simulink model "SMRsimplifiedmdl"  (R2020a)
settings: Solver=VariableStepAuto  StartTime=0.0  StopTime=10.0  RelTol=1e-3
settings Model: Creator=marce  LastModifiedBy=marce

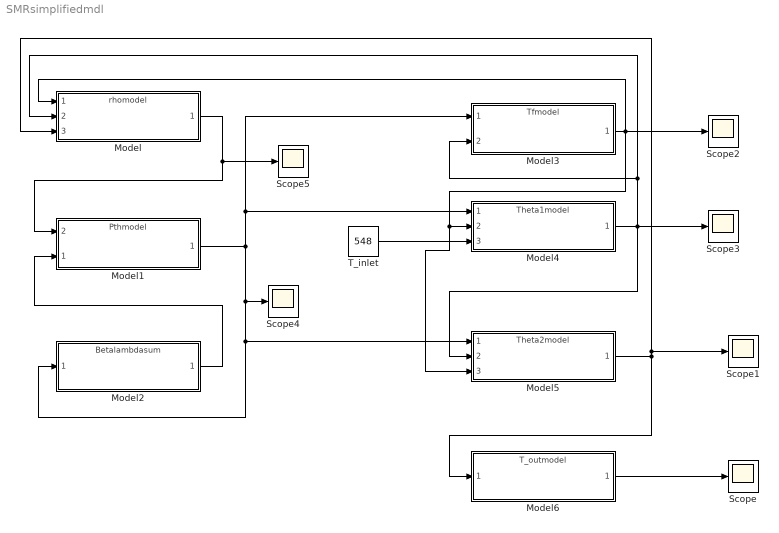
== system SMRsimplifiedmdl ==
  Model : ModelReference  ModelNameDialog=rhomodel.slx  SimulationMode=Normal  ModelReferenceVersion=1.1
  Model1 : ModelReference  ModelNameDialog=Pthmodel.slx  SimulationMode=Normal  ModelReferenceVersion=1.1
      settings: PortSchema="{\"entries\":[{\"content\":{\"sides\":[{\"content\":{\"connectorIds\":[\"In2\",\"In1\"]},\"type\":\"ConnectorPlacement.EquallySpacedRectSide\",\"uuid\":\"e3224459-0710-4ae8-912c-ffc24afd85fc\"},{\"content\":{\"connectorIds\":[\"Out1\"],\"side\":\"RIGHT\"},\"type\":\"ConnectorPlacement.EquallySpacedRectSide\",\"uuid\":\"0843270c-201a-4a4e-9d3a-b74d02db8142\"},{\"content\":{\"connectorIds\":[],\"side\":\"TOP\"},\"type\":\"ConnectorPlacement.EquallySpacedRectSide\",\"uuid\":\"bb3babb0-06ba-491a-a610-e4cb28426240\"}]},\"type\":\"ConnectorPlacement.EquallySpacedConnector\",\"uuid\":\"0ed36f46-bfee-4649-aea5-de7db864205e\"}],\"packageUris\":[\"http://schema.mathworks.com/mf0/Connector/19700101\"],\"version\":\"1.0\"}"
  Model2 : ModelReference  ModelNameDialog=Betalambdasum.slx  SimulationMode=Normal  ModelReferenceVersion=1.1
  Model3 : ModelReference  ModelNameDialog=Tfmodel.slx  SimulationMode=Normal  ModelReferenceVersion=1.2
  Model4 : ModelReference  ModelNameDialog=Theta1model.slx  SimulationMode=Normal  ModelReferenceVersion=1.2
  Model5 : ModelReference  ModelNameDialog=Theta2model.slx  SimulationMode=Normal  ModelReferenceVersion=1.2
  Model6 : ModelReference  ModelNameDialog=T_outmodel.slx  SimulationMode=Normal  ModelReferenceVersion=1.2
  Scope{,1..5} (6 alike) : Scope
  T_inlet : Constant  Value=548
  wires:
  Model2/1 -> Model1/1
  Model/1 -> Model1/2, Scope5/1
  Model1/1 -> Scope4/1, Model5/1, Model2/1, Model4/1, Model3/1
  Model4/1 -> Model5/2, Scope3/1, Model/2, Model3/2
  Model3/1 -> Model5/3, Model4/2, Scope2/1, Model/1
  Model5/1 -> Scope1/1, Model/3, Model6/1
  T_inlet/1 -> Model4/3
  Model6/1 -> Scope/1
